simulink model "part6"  (R2014a)
settings: Solver=ode45  StartTime=0.0  StopTime=10.0  RelTol=1e-3
settings Model: Creator=SuperUser  LastModifiedBy=SuperUser

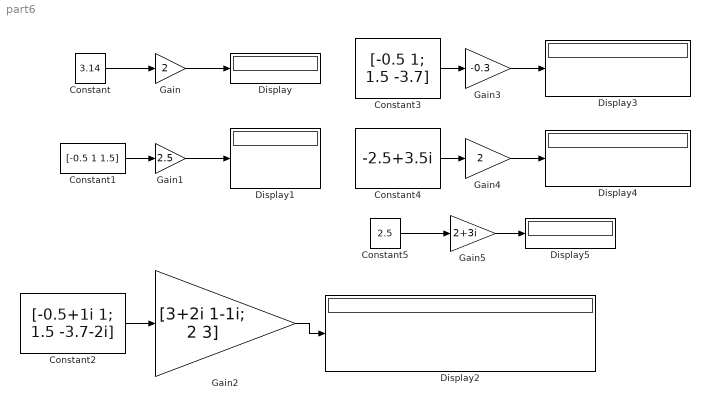
== system part6 ==
  Constant : Constant  Value=3.14
  Constant1 : Constant  Value=[-0.5 1 1.5]
  Constant2 : Constant  Value=[-0.5+1i 1; 1.5 -3.7-2i]
  Constant3 : Constant  Value=[-0.5 1; 1.5 -3.7]
  Constant4 : Constant  Value=-2.5+3.5i
  Constant5 : Constant  Value=2.5
  Display{,1..5} (6 alike) : Display
  Gain : Gain  Gain=2
  Gain1 : Gain  Gain=2.5
  Gain2 : Gain  Gain=[3+2i 1-1i; 2 3]
  Gain3 : Gain  Gain=-0.3
  Gain4 : Gain  Gain=2
  Gain5 : Gain  Gain=2+3i
  wires:
  Constant/1 -> Gain/1
  Gain/1 -> Display/1
  Constant1/1 -> Gain1/1
  Gain1/1 -> Display1/1
  Constant2/1 -> Gain2/1
  Gain2/1 -> Display2/1
  Constant3/1 -> Gain3/1
  Gain3/1 -> Display3/1
  Constant4/1 -> Gain4/1
  Gain4/1 -> Display4/1
  Constant5/1 -> Gain5/1
  Gain5/1 -> Display5/1
